simulink model "lab_3_conv_encoder_k3"  (Simulink 8.0)
settings: Solver=VariableStepDiscrete  StartTime=0.0  StopTime=0.00008  RelTol=1e-3
PreLoadFcn:
  | %-- Initialize myTrellis structure
  | myTrellis.numInputSymbols = 8;
  | myTrellis.numOutputSymbols = 16;
  | myTrellis.numStates = 8;
  | 
  | myTrellis.nextStates = [0     1     2     3     0     1     2     3;
  |                         6     7     4     5     6     7     4     5;
  |                         1     0     3     2     1     0     3     2;
  |                         7     6     5     4     7     6     5     4;
  |                         2     3     0     1     2     3     0     1;
  |                         4     5     6     7     4     5     6     7;
  |                         3     2     1     0     3     2     1     0;
  |                         5     4     7     6     5     4     7     6];
  | myTrellis.outputs =  [0     2     4     6    10    12    14    16;
  |                       1     3     5     7    11    13    15    17;
  |                       0     2     4     6    10    12    14    16;
  |                       1     3     5     7    11    13    15    17;
  |                       0     2     4     6    10    12    14    16;
  |                       1     3     5     7    11    13    15    17;
  |                       0     2     4     6    10    12    14    16;
  |                       1     3     5     7    11    13    15    17];
values from neighbouring files (symbols this model uses):
  Tb = 1/Rb    (= 1.11607142857e-06)    [lab_3_parameters.m]
libraries: dspsigops x3, commsink2 x2, commcnvcod2 x2, dspindex x2, commrandsrc2 x1
CloseFcn:
  | clear myTrellis convSigsOut;
settings Model: Creator=arodrigu  LastModifiedBy=yuw  BufferReuse=off
settings DataIOCC: SignalLoggingSaveFormat=ModelDataLogs  SaveOutput=off  SaveTime=off  SignalLoggingName=convSigsOut
settings OptimizationCC: BooleanDataType=off  InlineInvariantSignals=on  OptimizeBlockIOStorage=off  BufferReuse=off  ExpressionFolding=off  LocalBlockOutputs=off  InitFltsAndDblsToZero=on
settings DebuggingCC: SaveWithParameterizedLinksMsg=none  SignalResolutionControl=TryResolveAllWithWarning  SolverPrmCheckMsg=none  MultiTaskDSMMsg=warning  MultiTaskCondExecSysMsg=none  FcnCallInpInsideContextMsg=UseLocalSettings  StrictBusMsg=None
settings HardwareCC: ProdHWDeviceType=Specified
settings RTWCC: IncludeERTFirstTime=on
settings CodeAppCC: MangleLength=5
settings GRTTargetCC: TargetFcnLib=ansi_tfl_tmw.mat  CombineOutputUpdateFcns=off  GRTInterface=on

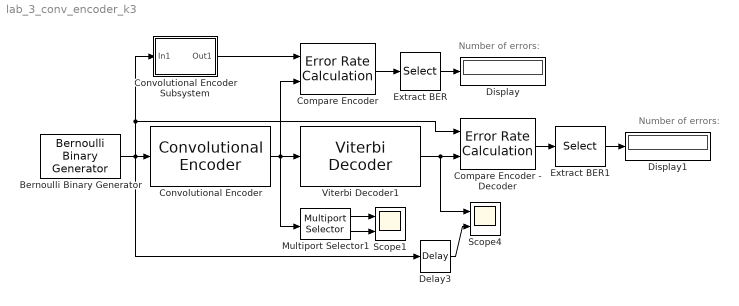
== system lab_3_conv_encoder_k3 ==
  note: Number of errors:
  note: Number of errors:
  Bernoulli Binary Generator : commrandsrc2/Bernoulli Binary Generator  P=0.5  seed=61  Ts=Tb  frameBased=on  sampPerFrame=1  orient=off  outDataType=double
  Compare Encoder - Decoder : commsink2/Error Rate Calculation  N=96  st_delay=0  cp_mode=Entire frame  subframe=[]  PMode=Port  WsName=ErrorVec  RsMode2=off  stop=off  numErr=100  maxBits=1e6
  Compare Encoder : commsink2/Error Rate Calculation  N=0  st_delay=0  cp_mode=Entire frame  subframe=[]  PMode=Port  WsName=ErrorVec  RsMode2=off  stop=off  numErr=100  maxBits=1e6
  Convolutional Encoder : commcnvcod2/Convolutional Encoder  trellis=poly2trellis(3, [6 7])  opMode=Continuous  DelayedResetAction=off  hasIniStPort=off  hasFinStPort=off  usePuncVector=off  punctureVector=[1; 1; 0; 1; 0; 1]  reset=Unused parameter value
  Convolutional Encoder Subsystem : Subsystem
  Delay3 : dspsigops/Delay  InputProcessing=Inherited (this choice will be removed - see release notes)  dly_unit=Samples  delay=96  ic_detail=off  dif_ic_for_ch=off  dif_ic_for_dly=off  ic=0  reset_popup=None
  Display : Display
  Display1 : Display
  Extract BER : Selector  InputPortWidth=3  IndexOptions=Index vector (dialog)  Indices=1  OutputSizes=1
  Extract BER1 : Selector  InputPortWidth=3  IndexOptions=Index vector (dialog)  Indices=1  OutputSizes=1
  Multiport Selector1 : dspindex/Multiport Selector  rowsOrCols=Rows  idxCellArray={1 2}  idxErrMode=Clip Index
  Scope1 : Scope  NumInputPorts=2
      settings: YMin=-5~-5  YMax=5~5
  Scope4 : Scope  NumInputPorts=2
      settings: YMin=-5~-5  YMax=5~5  SaveName=ScopeData4
  Viterbi Decoder1 : commcnvcod2/Viterbi Decoder  trellis=poly2trellis(3, [6 7])  isPunctured=off  punctureVector=[1; 1; 0; 1; 0; 1]  erasures=off  dectype=Hard decision  runSigValErrCheck=off  nsdecb=4  smWordLength=16  tbdepth=96  opmode=Continuous  reset=off  outDataType=double  delayedResetAction=off
  wires:
  Bernoulli Binary Generator/1 -> Convolutional Encoder/1, Delay3/1, Convolutional Encoder Subsystem/1(In1), Compare Encoder - Decoder/1
  Compare Encoder/1 -> Extract BER/1
  Extract BER/1 -> Display/1
  Convolutional Encoder/1 -> Multiport Selector1/1, Viterbi Decoder1/1, Compare Encoder/2
  Multiport Selector1/1 -> Scope1/1
  Multiport Selector1/2 -> Scope1/2
  Compare Encoder - Decoder/1 -> Extract BER1/1
  Extract BER1/1 -> Display1/1
  Viterbi Decoder1/1 -> Compare Encoder - Decoder/2, Scope4/1
  Delay3/1 -> Scope4/2
  Convolutional Encoder Subsystem/1(Out1) -> Compare Encoder/1

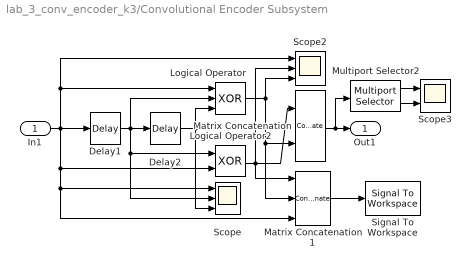
== system lab_3_conv_encoder_k3/Convolutional Encoder Subsystem ==
  In1 : Inport
  Delay1 : dspsigops/Delay  InputProcessing=Inherited (this choice will be removed - see release notes)  dly_unit=Samples  delay=1  ic_detail=off  dif_ic_for_ch=off  dif_ic_for_dly=off  ic=0  reset_popup=None
  Delay2 : dspsigops/Delay  InputProcessing=Inherited (this choice will be removed - see release notes)  dly_unit=Samples  delay=1  ic_detail=off  dif_ic_for_ch=off  dif_ic_for_dly=off  ic=0  reset_popup=None
  Logical Operator : Logic  Operator=XOR  Inputs=3  AllPortsSameDT=off
  Logical Operator2 : Logic  Operator=XOR  AllPortsSameDT=off
  Matrix Concatenation : Concatenate  Mode=Multidimensional array
  Matrix Concatenation1 : Concatenate  NumInputs=3  Mode=Multidimensional array  ConcatenateDimension=2
  Multiport Selector2 : dspindex/Multiport Selector  rowsOrCols=Rows  idxCellArray={1 2}  idxErrMode=Clip Index
  Scope : Scope  NumInputPorts=3
      settings: YMin=-5~-5~-5  YMax=5~5~5
  Scope2 : Scope  NumInputPorts=3
      settings: YMin=-5~-5~-5  YMax=5~5~5  SaveName=ScopeData2
  Scope3 : Scope  NumInputPorts=2
      settings: YMin=-5~-5  YMax=5~5  SaveName=ScopeData3
  Signal To Workspace : SignalToWorkspace  VariableName=In_Cod
      settings: CopyFcn=dspblkcopystw(gcbh);
  Out1 : Outport
  wires:
  Delay2/1 -> Logical Operator/3, Scope/3
  Delay1/1 -> Delay2/1, Logical Operator/2, Scope/2, Logical Operator2/1
  Multiport Selector2/1 -> Scope3/1
  Multiport Selector2/2 -> Scope3/2
  Logical Operator/1 -> Scope2/3, Matrix Concatenation/2, Matrix Concatenation1/2
  Logical Operator2/1 -> Scope2/2, Matrix Concatenation/1, Matrix Concatenation1/1
  In1/1 -> Delay1/1, Logical Operator2/2, Scope/1, Matrix Concatenation1/3, Logical Operator/1, Scope2/1
  Matrix Concatenation1/1 -> Signal To Workspace/1
  Matrix Concatenation/1 -> Out1/1, Multiport Selector2/1
